simulink model "Simulation"  (R2023b)
settings: Solver=FixedStepAuto  StartTime=0.0  StopTime=200  FixedStep=1e-4  RelTol=1e-3
model workspace (MAT data in the model file):
  Kp = 3.0773
  Td = 9.113
  Ti = 0.240894199268
settings Model: Creator=Son  LastModifiedBy=Son

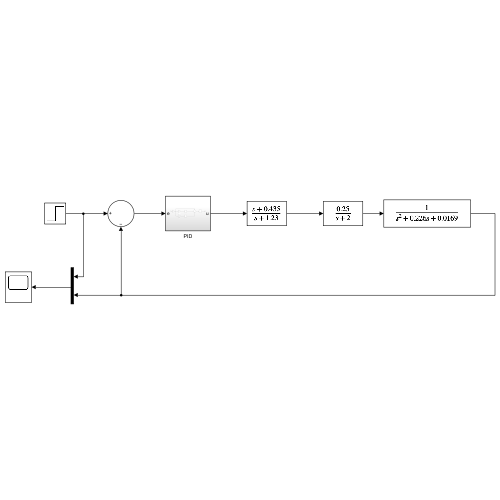
[thumbnail: Simulink's stored preview of the top-level diagram]
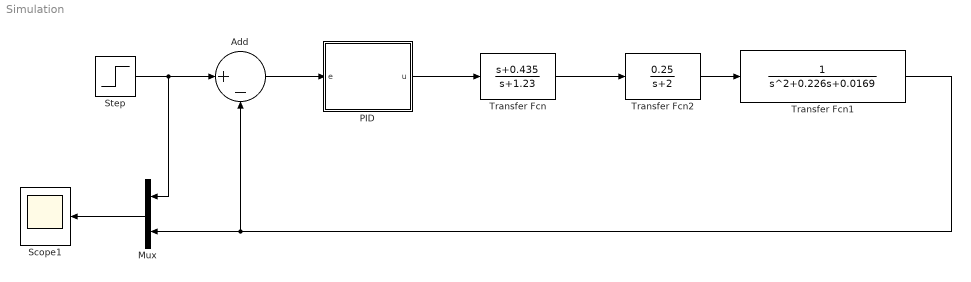
== system Simulation ==
  Add : Sum  Inputs=|+-
  Mux : Mux  Inputs=2
  PID : Subsystem
  Scope1 : Scope
  Step : Step  SampleTime=0
  Transfer Fcn : TransferFcn  Numerator=[1 0.435]  Denominator=[1 1.23]
  Transfer Fcn1 : TransferFcn  Denominator=[1 0.226 0.0169]
  Transfer Fcn2 : TransferFcn  Numerator=[0.25]  Denominator=[1 2]
  wires:
  Transfer Fcn/1 -> Transfer Fcn2/1
  Transfer Fcn2/1 -> Transfer Fcn1/1
  Transfer Fcn1/1 -> Mux/2, Add/2
  Step/1 -> Mux/1, Add/1
  Mux/1 -> Scope1/1
  Add/1 -> PID/1(e)
  PID/1(u) -> Transfer Fcn/1

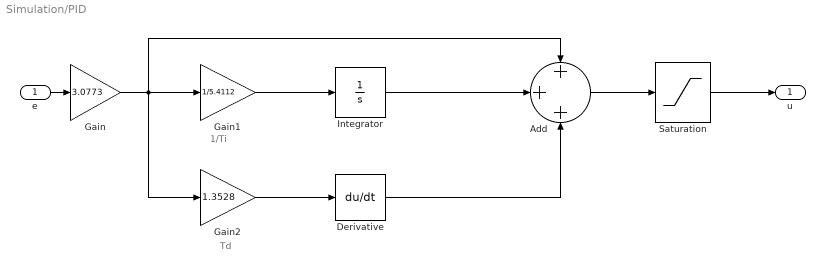
== system Simulation/PID ==
  note: Td
  note: 1/Ti
  e : Inport
  Add : Sum  Inputs=+++
  Derivative : Derivative
  Gain : Gain  Gain=3.0773
  Gain1 : Gain  Gain=1/5.4112
  Gain2 : Gain  Gain=1.3528
  Integrator : Integrator
  Saturation : Saturate  UpperLimit=100  LowerLimit=-100
  u : Outport
  wires:
  Gain1/1 -> Integrator/1
  Derivative/1 -> Add/3
  Gain2/1 -> Derivative/1
  Integrator/1 -> Add/2
  e/1 -> Gain/1
  Add/1 -> Saturation/1
  Saturation/1 -> u/1
  Gain/1 -> Add/1, Gain1/1, Gain2/1
